simulink model "sim_DecouplingPID_R2012a"  (Simulink 7.9)
settings: Solver=ode45  StartTime=0.0  StopTime=180  RelTol=1e-3
undefined symbols (not defined in the file): KPID
libraries: simulink x2, lib_Lagrangian_Model_Nonlinear x1
settings Model: Creator=ottoe  LastModifiedBy=ottoe  CovModelRefEnable=off
settings DataIOCC: LimitDataPoints=off  SaveFormat=StructureWithTime  SignalLoggingSaveFormat=Dataset
settings OptimizationCC: ExpressionDepthLimit=128
settings DebuggingCC: UnderspecifiedInitializationDetection=Simplified  MergeDetectMultiDrivingBlocksExec=error  SolverPrmCheckMsg=none  FrameProcessingCompatibilityMsg=error  StateNameClashWarn=none
settings HardwareCC: ProdBitPerPointer=64  ProdLargestAtomicFloat=Float  ProdIntDivRoundTo=Zero  ProdEndianess=LittleEndian  ProdHWDeviceType=Specified
settings ModelReferenceCC: PropagateSignalLabelsOutOfModel=on
settings CodeAppCC: CustomSymbolStrType=$N$R$M_T
settings GRTTargetCC: CodeReplacementLibrary=C89/C90 (ANSI)

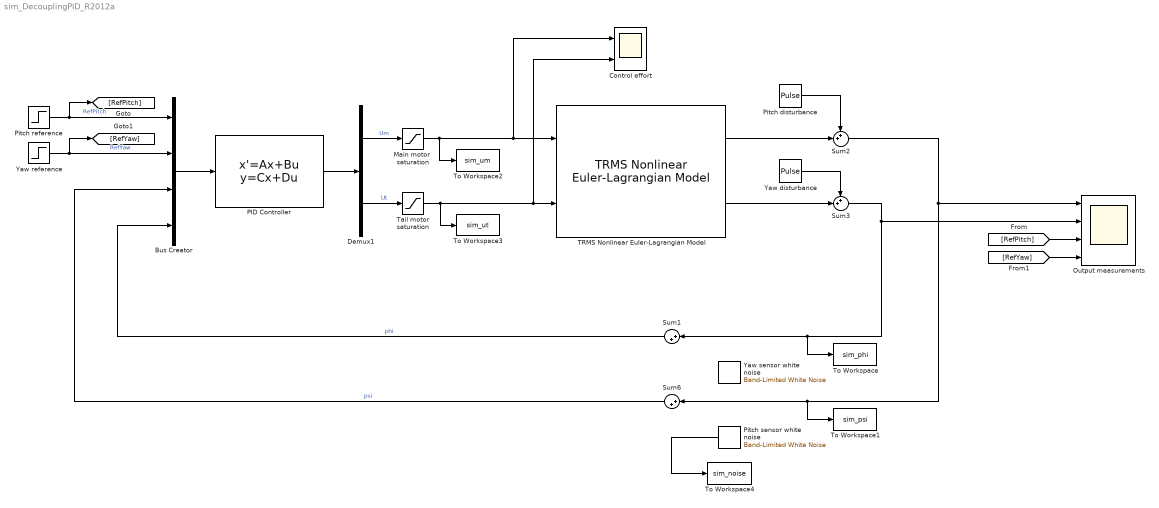
== system sim_DecouplingPID_R2012a ==
  Bus Creator : BusCreator  Inputs=4
  Control effort : Scope  NumInputPorts=2
      settings: TimeRange=auto  ShowLegends=on  MaxDataPoints=5000  SaveToWorkspace=off  YMin=-3.125~-5  YMax=3.125~5  SampleTime=-1
  Demux1 : Demux  Outputs=2
  Main motor  saturation : Saturate  UpperLimit=2.5  LowerLimit=-2.5
  Output measurements : Scope  NumInputPorts=4
      settings: TimeRange=auto  ShowLegends=on  MaxDataPoints=5000  SaveToWorkspace=off  YMin=-1.40106~-5~-5~-5  YMax=0.37256~5~5~5  SampleTime=-1
  PID Controller : StateSpace  A=KPID.A  B=KPID.B  C=KPID.C  D=KPID.D  X0=0
  Pitch disturbance : DiscretePulseGenerator  PulseType=Time based  Amplitude=0.1  Period=100  PulseWidth=0.1  PhaseDelay=80
  Pitch reference : Step  Time=100  After=0  SampleTime=0
  Pitch sensor white noise : simulink/Sources/Band-Limited White Noise  Cov=[0.000000001]  Ts=0.001  seed=[23341]
  Sum1 : Sum  Inputs=|++
  Sum2 : Sum  Inputs=++|
  Sum3 : Sum  Inputs=++|
  Sum6 : Sum  Inputs=|++
  TRMS Nonlinear Euler-Lagrangian Model : lib_Lagrangian_Model_Nonlinear/TRMS Nonlinear Euler-Lagrangian Model  Psi_zero=0  Psi_dot_zero=0  Phi_zero=0  Phi_dot_zero=0  Wm_zero=0  Wt_zero=0
  Tail motor saturation : Saturate  UpperLimit=2.5  LowerLimit=-2.5
  To Workspace : ToWorkspace  VariableName=sim_phi  SaveFormat=Timeseries  SampleTime=-1
  To Workspace1 : ToWorkspace  VariableName=sim_psi  SaveFormat=Timeseries  SampleTime=-1
  To Workspace2 : ToWorkspace  VariableName=sim_um  SaveFormat=Timeseries  SampleTime=-1
  To Workspace3 : ToWorkspace  VariableName=sim_ut  SaveFormat=Timeseries  SampleTime=-1
  To Workspace4 : ToWorkspace  VariableName=sim_noise  SaveFormat=Timeseries  SampleTime=-1
  Yaw disturbance : DiscretePulseGenerator  PulseType=Time based  Amplitude=0.1  Period=100  PulseWidth=0.1  PhaseDelay=120
  Yaw reference : Step  Time=140  After=0  SampleTime=0
  Yaw sensor white noise : simulink/Sources/Band-Limited White Noise  Cov=[0.000000001]  Ts=0.001  seed=[23341]
  wires:
  Bus Creator/1 -> PID Controller/1
  PID Controller/1 -> Demux1/1
  Demux1/1 -> Main motor  saturation/1  "Um"
  Demux1/2 -> Tail motor saturation/1  "Ut"
  Pitch reference/1 -> [RefPitch], Bus Creator/1  "RefPitch"
  Yaw reference/1 -> [RefYaw], Bus Creator/2  "RefYaw"
  Tail motor saturation/1 -> To Workspace3/1, TRMS Nonlinear Euler-Lagrangian Model/2, Control effort/2
  Sum6/1 -> Bus Creator/3  "psi"
  Sum1/1 -> Bus Creator/4  "phi"
  TRMS Nonlinear Euler-Lagrangian Model/1 -> Sum2/2
  TRMS Nonlinear Euler-Lagrangian Model/2 -> Sum3/2
  Pitch disturbance/1 -> Sum2/1
  Yaw disturbance/1 -> Sum3/1
  Main motor  saturation/1 -> To Workspace2/1, Control effort/1, TRMS Nonlinear Euler-Lagrangian Model/1
  Sum3/1 -> Output measurements/2, To Workspace/1, Sum1/1
  Sum2/1 -> Output measurements/1, To Workspace1/1, Sum6/1
  Pitch sensor white noise/1 -> To Workspace4/1
  [RefPitch] -> Output measurements/3
  [RefYaw] -> Output measurements/4
